simulink model "simulink_kaskada_dva"  (R2015a)
settings: Solver=FixedStepDiscrete  StartTime=0.0  StopTime=99.0  FixedStep=1  RelTol=1e-3
settings Model: Creator=Bojana Vasic  LastModifiedBy=Bojana Vasic

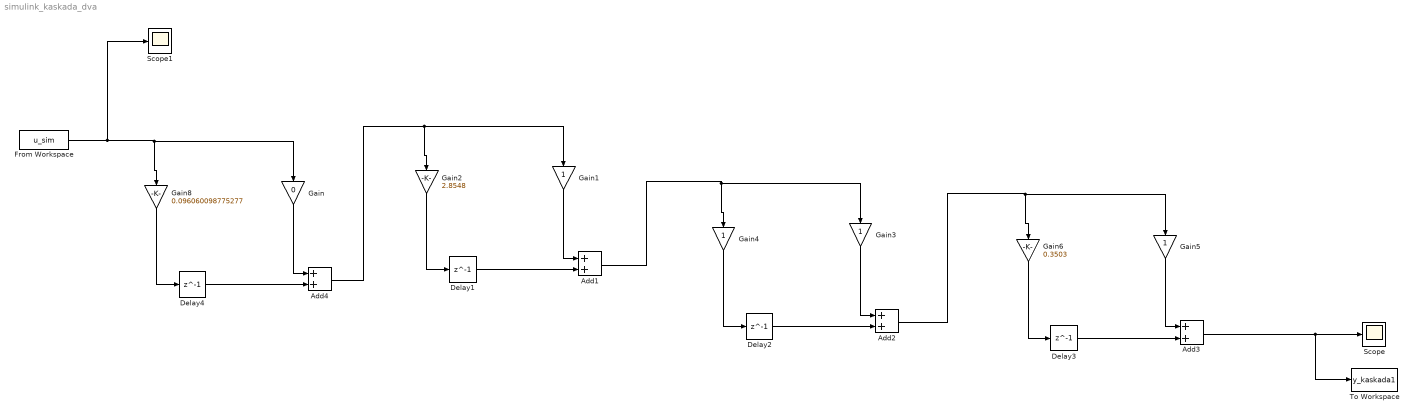
== system simulink_kaskada_dva ==
  Add{1..4} (4 alike) : Sum
  Delay{1..4} (4 alike) : Delay  DelayLength=1
  From Workspace : FromWorkspace  VariableName=u_sim  SampleTime=1
  Gain : Gain  Gain=0
  Gain{1,3..5} (4 alike) : Gain
  Gain2 : Gain  Gain=2.8548
  Gain6 : Gain  Gain=0.3503
  Gain8 : Gain  Gain=0.096060098775277
  Scope : Scope
  Scope1 : Scope
  To Workspace : ToWorkspace  VariableName=y_kaskada1  SampleTime=-1
      settings: Save2DSignal=2-D array (concatenate along first dimension)
  wires:
  From Workspace/1 -> Gain/1, Gain8/1, Scope1/1
  Gain/1 -> Add4/1
  Gain8/1 -> Delay4/1
  Delay4/1 -> Add4/2
  Add4/1 -> Gain1/1, Gain2/1
  Gain1/1 -> Add1/1
  Gain2/1 -> Delay1/1
  Delay1/1 -> Add1/2
  Add1/1 -> Gain3/1, Gain4/1
  Gain3/1 -> Add2/1
  Gain4/1 -> Delay2/1
  Delay2/1 -> Add2/2
  Add2/1 -> Gain5/1, Gain6/1
  Gain5/1 -> Add3/1
  Gain6/1 -> Delay3/1
  Delay3/1 -> Add3/2
  Add3/1 -> To Workspace/1, Scope/1
